simulink model "adapt"  (Simulink 7.9)
settings: Solver=ode45  StartTime=0.0  StopTime=100  RelTol=1e-3
settings Model: Creator=Floater  LastModifiedBy=jdenil
settings OptimizationCC: InlineParams=on  InitFltsAndDblsToZero=on
settings DebuggingCC: FcnCallInpInsideContextMsg=Use local settings  StrictBusMsg=Warning
settings GRTTargetCC: CombineOutputUpdateFcns=off  GRTInterface=on

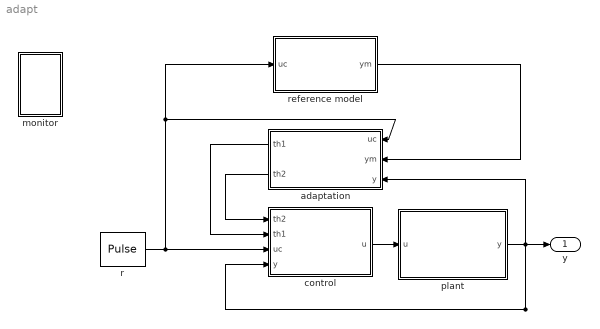
== system adapt ==
  adaptation : Subsystem
  control : Subsystem
  monitor : Subsystem
  plant : Subsystem
  r : DiscretePulseGenerator  PulseType=Time based  Period=20  PulseWidth=50
  reference model : Subsystem
  y : Outport
  wires:
  r/1 -> reference model/1(uc), adaptation/1(uc), control/3(uc)
  control/1(u) -> plant/1(u)
  reference model/1(ym) -> adaptation/2(ym)
  plant/1(y) -> control/4(y), adaptation/3(y), y/1
  adaptation/1(th1) -> control/2(th1)
  adaptation/2(th2) -> control/1(th2)

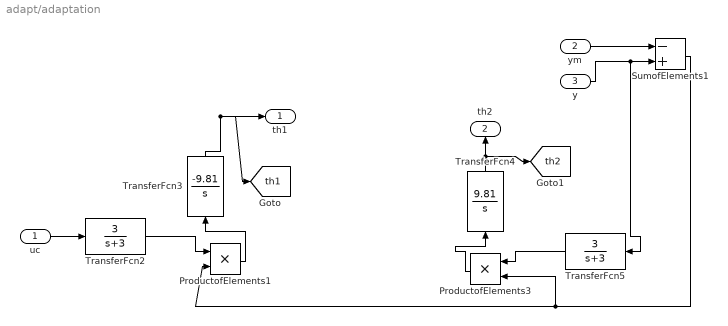
== system adapt/adaptation ==
  uc : Inport
  ym : Inport  Port=2
  y : Inport  Port=3
  ProductofElements1 : Product  Inputs=**
  ProductofElements3 : Product  Inputs=**
  SumofElements1 : Sum  Inputs=-+
  TransferFcn2 : TransferFcn  Numerator=[3]  Denominator=[1 3]
  TransferFcn3 : TransferFcn  Numerator=[-9.81]  Denominator=[1 0]
  TransferFcn4 : TransferFcn  Numerator=[9.81]  Denominator=[1 0]
  TransferFcn5 : TransferFcn  Numerator=[3]  Denominator=[1 3]
  th1 : Outport
  th2 : Outport  Port=2
  tag scope: th1=global, th2=global
  wires:
  TransferFcn2/1 -> ProductofElements1/1
  ProductofElements1/1 -> TransferFcn3/1
  TransferFcn3/1 -> [th1], th1/1
  TransferFcn4/1 -> [th2], th2/1
  ProductofElements3/1 -> TransferFcn4/1
  TransferFcn5/1 -> ProductofElements3/1
  SumofElements1/1 -> ProductofElements1/2, ProductofElements3/2
  y/1 -> SumofElements1/2, TransferFcn5/1
  uc/1 -> TransferFcn2/1
  ym/1 -> SumofElements1/1

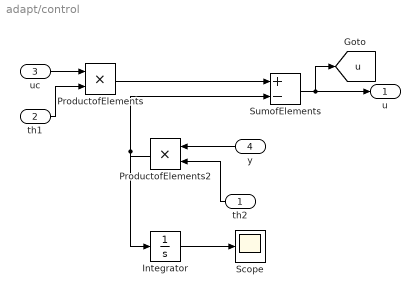
== system adapt/control ==
  th2 : Inport
  th1 : Inport  Port=2
  uc : Inport  Port=3
      settings: AttributesFormatString=%<Port>
  y : Inport  Port=4
  Integrator : Integrator
  ProductofElements : Product  Inputs=**
  ProductofElements2 : Product  Inputs=**
  Scope : Scope
      settings: SaveName=ScopeData2
  SumofElements : Sum  Inputs=+-
  u : Outport
  tag scope: u=global
  wires:
  ProductofElements/1 -> SumofElements/1
  ProductofElements2/1 -> Integrator/1, SumofElements/2
  uc/1 -> ProductofElements/1
  th1/1 -> ProductofElements/2
  y/1 -> ProductofElements2/1
  th2/1 -> ProductofElements2/2
  SumofElements/1 -> u/1, [u]
  Integrator/1 -> Scope/1

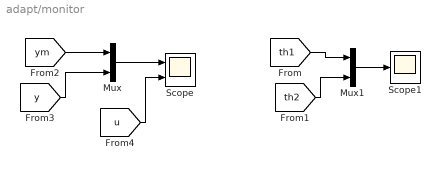
== system adapt/monitor ==
  Mux : Mux  Inputs=2
  Mux1 : Mux  Inputs=2
  Scope : Scope  NumInputPorts=2
      settings: TimeRange=100  YMin=0~-0.5  YMax=1.4~2.5
  Scope1 : Scope
      settings: TimeRange=100  YMin=-0.5  YMax=3
  wires:
  Mux/1 -> Scope/1
  Mux1/1 -> Scope1/1
  [th1] -> Mux1/1
  [th2] -> Mux1/2
  [ym] -> Mux/1
  [y] -> Mux/2
  [u] -> Scope/2

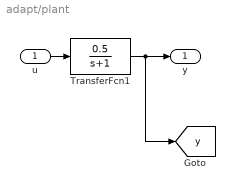
== system adapt/plant ==
  u : Inport
  TransferFcn1 : TransferFcn  Numerator=[0.5]  Denominator=[1 1]
  y : Outport
  tag scope: y=global
  wires:
  u/1 -> TransferFcn1/1
  TransferFcn1/1 -> y/1, [y]

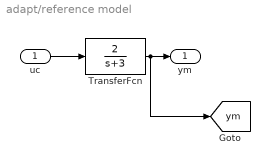
== system adapt/reference model ==
  uc : Inport
  TransferFcn : TransferFcn  Numerator=[2]  Denominator=[1 3]
  ym : Outport
  tag scope: ym=global
  wires:
  uc/1 -> TransferFcn/1
  TransferFcn/1 -> ym/1, [ym]
